simulink model "FOG_v1"  (R2023b)
settings: Solver=ode4  StartTime=0.0  StopTime=0.05  FixedStep=1e-6  RelTol=1e-3
undefined symbols (not defined in the file): beta, f_mod, fc_lp, K_norm, K_phase_to_deg, K_sag, Omega_deg_s, Pscale, Rpd, Rtia, visibility
settings Model: Creator=molik  LastModifiedBy=molik

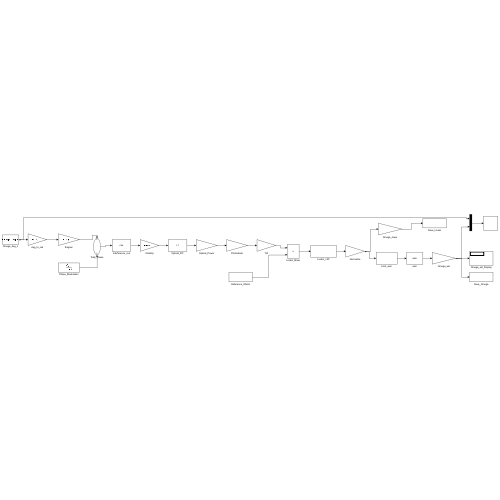
[thumbnail: Simulink's stored preview of the top-level diagram]
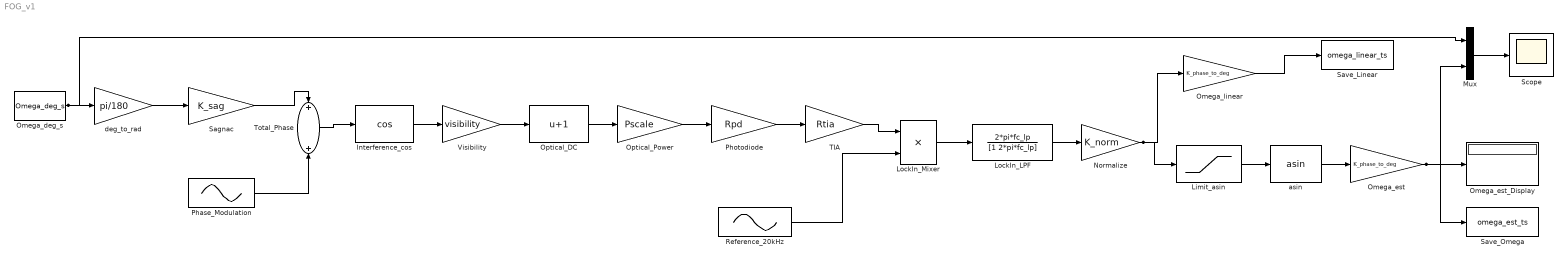
== system FOG_v1 ==
  Interference_cos : Trigonometry  Operator=cos
  Limit_asin : Saturate  UpperLimit=0.999999  LowerLimit=-0.999999
  LockIn_LPF : TransferFcn  Numerator=2*pi*fc_lp  Denominator=[1 2*pi*fc_lp]
  LockIn_Mixer : Product
  Mux : Mux  Inputs=2
  Normalize : Gain  Gain=K_norm
  Omega_deg_s : Constant  Value=Omega_deg_s
  Omega_est : Gain  Gain=K_phase_to_deg
  Omega_est_Display : Display
  Omega_linear : Gain  Gain=K_phase_to_deg
  Optical_DC : Bias  Bias=1  SaturateOnIntegerOverflow=off
  Optical_Power : Gain  Gain=Pscale
  Phase_Modulation : Sin  Amplitude=beta  Frequency=2*pi*f_mod  SampleTime=0
  Photodiode : Gain  Gain=Rpd
  Reference_20kHz : Sin  Frequency=2*pi*f_mod  SampleTime=0
  Sagnac : Gain  Gain=K_sag
  Save_Linear : ToWorkspace  VariableName=omega_linear_ts  SaveFormat=Timeseries  SampleTime=-1
  Save_Omega : ToWorkspace  VariableName=omega_est_ts  SaveFormat=Timeseries  SampleTime=-1
  Scope : Scope
  TIA : Gain  Gain=Rtia
  Total_Phase : Sum
  Visibility : Gain  Gain=visibility
  asin : Trigonometry  Operator=asin
  deg_to_rad : Gain  Gain=pi/180
  wires:
  Omega_deg_s/1 -> deg_to_rad/1, Mux/1
  deg_to_rad/1 -> Sagnac/1
  Sagnac/1 -> Total_Phase/1
  Phase_Modulation/1 -> Total_Phase/2
  Total_Phase/1 -> Interference_cos/1
  Interference_cos/1 -> Visibility/1
  Visibility/1 -> Optical_DC/1
  Optical_DC/1 -> Optical_Power/1
  Optical_Power/1 -> Photodiode/1
  Photodiode/1 -> TIA/1
  TIA/1 -> LockIn_Mixer/1
  Reference_20kHz/1 -> LockIn_Mixer/2
  LockIn_Mixer/1 -> LockIn_LPF/1
  LockIn_LPF/1 -> Normalize/1
  Normalize/1 -> Omega_linear/1, Limit_asin/1
  Limit_asin/1 -> asin/1
  asin/1 -> Omega_est/1
  Omega_est/1 -> Omega_est_Display/1, Save_Omega/1, Mux/2
  Omega_linear/1 -> Save_Linear/1
  Mux/1 -> Scope/1
